simulink model "partial_product"  (Simulink 8.0)
settings: Solver=ode45  StartTime=0.0  StopTime=10.0  RelTol=1e-3
settings Model: Creator=glyme  LastModifiedBy=dell
settings DataIOCC: SignalLoggingSaveFormat=ModelDataLogs
settings DebuggingCC: FcnCallInpInsideContextMsg=EnableAllAsWarning

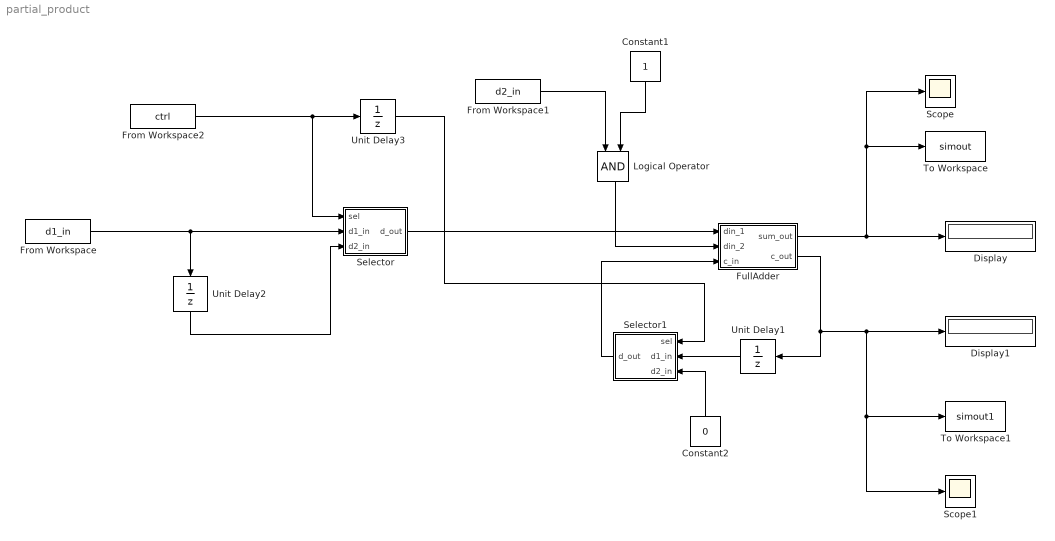
== system partial_product ==
  Constant1 : Constant  OutDataTypeStr=boolean
  Constant2 : Constant  Value=0  OutDataTypeStr=boolean
  Display : Display
  Display1 : Display
  From Workspace : FromWorkspace  VariableName=d1_in  OutDataTypeStr=boolean  SampleTime=1
  From Workspace1 : FromWorkspace  VariableName=d2_in  OutDataTypeStr=boolean  SampleTime=1
  From Workspace2 : FromWorkspace  VariableName=ctrl  OutDataTypeStr=boolean  SampleTime=1
  FullAdder : Subsystem
  Logical Operator : Logic  AllPortsSameDT=off  OutDataTypeStr=boolean
  Scope : Scope
  Scope1 : Scope
  Selector : Subsystem
  Selector1 : Subsystem
  To Workspace : ToWorkspace  VariableName=simout  SampleTime=1  SaveFormat=Timeseries
  To Workspace1 : ToWorkspace  VariableName=simout1  SampleTime=1  SaveFormat=Timeseries
  Unit Delay1 : UnitDelay
  Unit Delay2 : UnitDelay
  Unit Delay3 : UnitDelay
  wires:
  FullAdder/2(c_out) -> Scope1/1, To Workspace1/1, Display1/1, Unit Delay1/1
  Constant1/1 -> Logical Operator/2
  From Workspace2/1 -> Unit Delay3/1, Selector/1(sel)
  From Workspace/1 -> Selector/2(d1_in), Unit Delay2/1
  Unit Delay2/1 -> Selector/3(d2_in)
  From Workspace1/1 -> Logical Operator/1
  Logical Operator/1 -> FullAdder/2(din_2)
  Selector/1(d_out) -> FullAdder/1(din_1)
  FullAdder/1(sum_out) -> Scope/1, To Workspace/1, Display/1
  Unit Delay1/1 -> Selector1/2(d1_in)
  Constant2/1 -> Selector1/3(d2_in)
  Unit Delay3/1 -> Selector1/1(sel)
  Selector1/1(d_out) -> FullAdder/3(c_in)

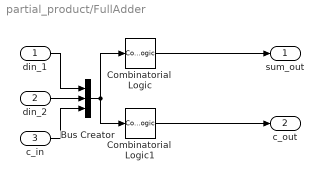
== system partial_product/FullAdder ==
  din_1 : Inport  OutDataTypeStr=boolean
  din_2 : Inport  Port=2  OutDataTypeStr=boolean
  c_in : Inport  Port=3  OutDataTypeStr=boolean
  Bus Creator : BusCreator  Inputs=3
  Combinatorial  Logic : CombinatorialLogic  TruthTable=[0;1;1;0;1;0;0;1]
  Combinatorial  Logic1 : CombinatorialLogic  TruthTable=[0;0;0;1;0;1;1;1]
  sum_out : Outport
  c_out : Outport  Port=2
  wires:
  Combinatorial  Logic/1 -> sum_out/1
  din_1/1 -> Bus Creator/1
  din_2/1 -> Bus Creator/2
  c_in/1 -> Bus Creator/3
  Bus Creator/1 -> Combinatorial  Logic/1, Combinatorial  Logic1/1
  Combinatorial  Logic1/1 -> c_out/1

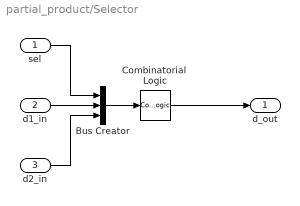
== system partial_product/Selector ==
  sel : Inport
  d1_in : Inport  Port=2
  d2_in : Inport  Port=3
  Bus Creator : BusCreator  Inputs=3
  Combinatorial  Logic : CombinatorialLogic  TruthTable=[0;0;1;1;0;1;0;1]
  d_out : Outport
  wires:
  sel/1 -> Bus Creator/1
  d1_in/1 -> Bus Creator/2
  d2_in/1 -> Bus Creator/3
  Bus Creator/1 -> Combinatorial  Logic/1
  Combinatorial  Logic/1 -> d_out/1

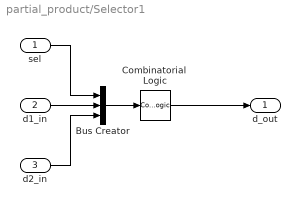
== system partial_product/Selector1 ==
  sel : Inport
  d1_in : Inport  Port=2
  d2_in : Inport  Port=3
  Bus Creator : BusCreator  Inputs=3
  Combinatorial  Logic : CombinatorialLogic  TruthTable=[0;0;1;1;0;1;0;1]
  d_out : Outport
  wires:
  sel/1 -> Bus Creator/1
  d1_in/1 -> Bus Creator/2
  d2_in/1 -> Bus Creator/3
  Bus Creator/1 -> Combinatorial  Logic/1
  Combinatorial  Logic/1 -> d_out/1
